simulink model "model"  (R2025b)
settings: Solver=ode1  StartTime=0.0  StopTime=Tstop  FixedStep=dt  RelTol=1e-3
undefined symbols (not defined in the file): d, N, opt_strategy, v0_vec, x0_vec
settings Model: Creator=Filippo  LastModifiedBy=dorec
settings DataIOCC: ReturnWorkspaceOutputs=off

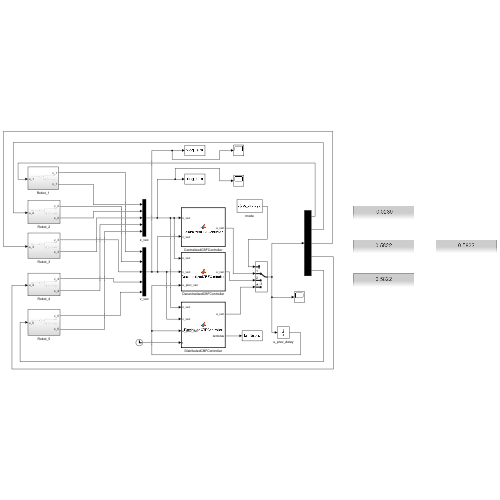
[thumbnail: Simulink's stored preview of the top-level diagram]
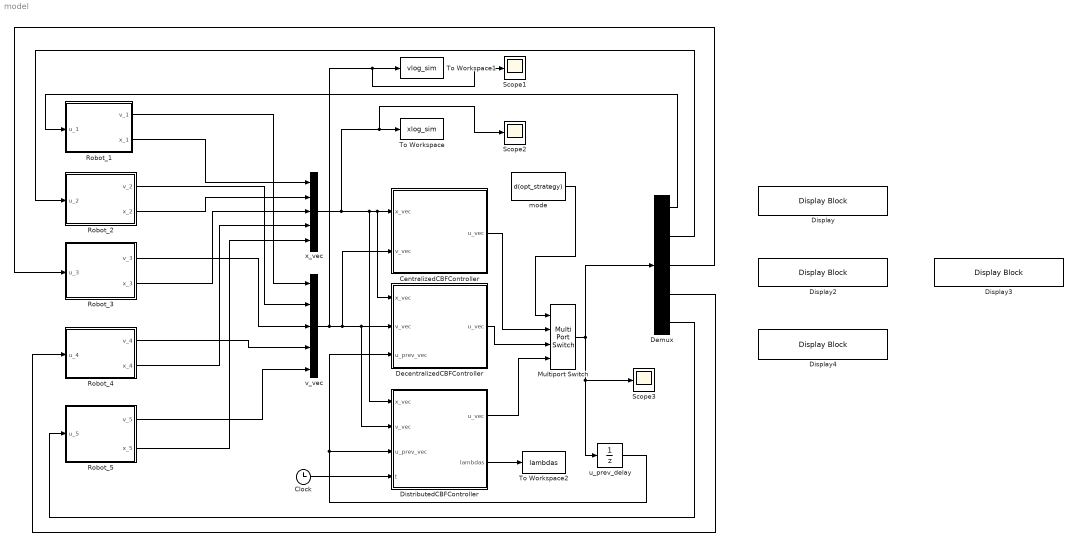
== system model ==
  CentralizedCBFController : MATLAB Function  TreatAsAtomicUnit=on
  Clock : Clock
  DecentralizedCBFController : MATLAB Function  TreatAsAtomicUnit=on
  Demux : Demux  Outputs=5
  Display{,2..4} (4 alike) : DisplayBlock  LabelPosition=Hide  Transparency=1  GridColor=[0.502, 0.502, 0.502]
  DistributedCBFController : MATLAB Function  TreatAsAtomicUnit=on
  Multiport Switch : MultiPortSwitch  SaturateOnIntegerOverflow=off  InputSameDT=off
  Robot_1 : Subsystem
  Robot_2 : Subsystem
  Robot_3 : Subsystem
  Robot_4 : Subsystem
  Robot_5 : Subsystem
  Scope1 : Scope
      settings: ActiveDisplayYMinimum=-1  ActiveDisplayYMaximum=1
  Scope2 : Scope
      settings: ActiveDisplayYMinimum=-11.952015322164979  ActiveDisplayYMaximum=12.436191131524438  DataLoggingVariableName=ScopeData2
  Scope3 : Scope
      settings: ActiveDisplayYMinimum=-11.952015322164979  ActiveDisplayYMaximum=12.436191131524438
  To Workspace : ToWorkspace  VariableName=xlog_sim  SampleTime=-1
  To Workspace1 : ToWorkspace  VariableName=vlog_sim  SampleTime=-1
  To Workspace2 : ToWorkspace  VariableName=lambdas  SampleTime=-1
  mode : Constant  Value=d(opt_strategy)
  u_prev_delay : UnitDelay  InitialCondition=zeros(2*N,1)  SampleTime=-1  HasFrameUpgradeWarning=on
  v_vec : Mux  Inputs=5
  x_vec : Mux  Inputs=5
  wires:
  CentralizedCBFController/1(u_vec) -> Multiport Switch/2
  u_prev_delay/1 -> DecentralizedCBFController/3(u_prev_vec), DistributedCBFController/3(u_prev_vec)
  mode/1 -> Multiport Switch/1
  Multiport Switch/1 -> Demux/1, Scope3/1, u_prev_delay/1
  DecentralizedCBFController/1(u_vec) -> Multiport Switch/3
  Robot_1/2(x_1) -> x_vec/1
  Robot_2/2(x_2) -> x_vec/2
  Robot_3/2(x_3) -> x_vec/3
  Robot_4/2(x_4) -> x_vec/4
  Robot_5/2(x_5) -> x_vec/5
  Robot_1/1(v_1) -> v_vec/1
  Robot_2/1(v_2) -> v_vec/2
  Robot_3/1(v_3) -> v_vec/3
  Robot_4/1(v_4) -> v_vec/4
  Robot_5/1(v_5) -> v_vec/5
  x_vec/1 -> Scope2/1, To Workspace/1, DistributedCBFController/1(x_vec), DecentralizedCBFController/1(x_vec), CentralizedCBFController/1(x_vec)
  v_vec/1 -> Scope1/1, To Workspace1/1, CentralizedCBFController/2(v_vec), DecentralizedCBFController/2(v_vec), DistributedCBFController/2(v_vec)
  Demux/5 -> Robot_5/1(u_5)
  Demux/1 -> Robot_1/1(u_1)
  Demux/4 -> Robot_4/1(u_4)
  Demux/3 -> Robot_3/1(u_3)
  Demux/2 -> Robot_2/1(u_2)
  Clock/1 -> DistributedCBFController/4(t)
  DistributedCBFController/1(u_vec) -> Multiport Switch/4
  DistributedCBFController/2(lambdas) -> To Workspace2/1

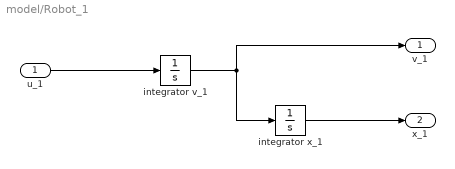
== system model/Robot_1 ==
  u_1 : Inport
  integrator v_1 : Integrator  InitialCondition=v0_vec(1:2)
  integrator x_1 : Integrator  InitialCondition=x0_vec(1:2)
  v_1 : Outport
  x_1 : Outport  Port=2
  wires:
  integrator v_1/1 -> v_1/1, integrator x_1/1
  u_1/1 -> integrator v_1/1
  integrator x_1/1 -> x_1/1

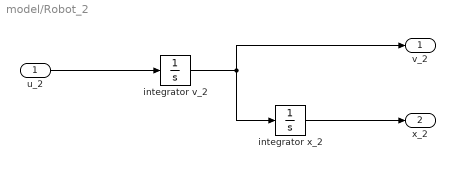
== system model/Robot_2 ==
  u_2 : Inport
  integrator v_2 : Integrator  InitialCondition=v0_vec(3:4)
  integrator x_2 : Integrator  InitialCondition=x0_vec(3:4)
  v_2 : Outport
  x_2 : Outport  Port=2
  wires:
  integrator v_2/1 -> v_2/1, integrator x_2/1
  u_2/1 -> integrator v_2/1
  integrator x_2/1 -> x_2/1

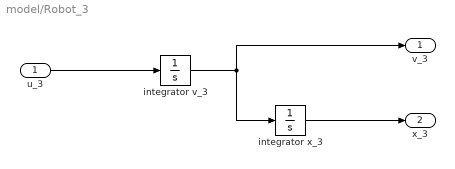
== system model/Robot_3 ==
  u_3 : Inport
  integrator v_3 : Integrator  InitialCondition=v0_vec(5:6)
  integrator x_3 : Integrator  InitialCondition=x0_vec(5:6)
  v_3 : Outport
  x_3 : Outport  Port=2
  wires:
  integrator v_3/1 -> v_3/1, integrator x_3/1
  u_3/1 -> integrator v_3/1
  integrator x_3/1 -> x_3/1

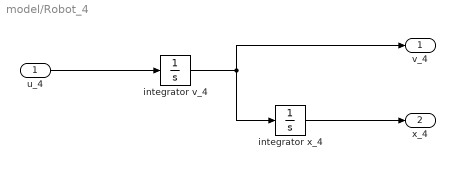
== system model/Robot_4 ==
  u_4 : Inport
  integrator v_4 : Integrator  InitialCondition=v0_vec(7:8)
  integrator x_4 : Integrator  InitialCondition=x0_vec(7:8)
  v_4 : Outport
  x_4 : Outport  Port=2
  wires:
  integrator v_4/1 -> v_4/1, integrator x_4/1
  u_4/1 -> integrator v_4/1
  integrator x_4/1 -> x_4/1

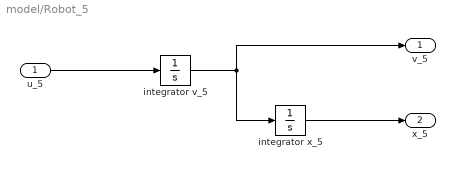
== system model/Robot_5 ==
  u_5 : Inport
  integrator v_5 : Integrator  InitialCondition=v0_vec(9:10)
  integrator x_5 : Integrator  InitialCondition=x0_vec(9:10)
  v_5 : Outport
  x_5 : Outport  Port=2
  wires:
  integrator v_5/1 -> v_5/1, integrator x_5/1
  u_5/1 -> integrator v_5/1
  integrator x_5/1 -> x_5/1

== matlab function model/DecentralizedCBFController ==
  data: x_vec input; u_vec output; v_vec input; u_prev_vec input
function u_vec = DecentralizedCBFController(x_vec, v_vec, u_prev_vec)
%#codegen
% Wrapper per chiamare decentralized_cbf_step da Simulink

coder.extrinsic('decentralized_cbf_step');

% Numero agenti (qui puoi fissare N=5 o leggere dal base workspace)
N = 5;                     % oppure usa evalin se vuoi:
% coder.extrinsic('evalin');
% N = evalin('base','N');

u_vec = zeros(2*N,1);      % per inferenza dimensioni

u_vec = decentralized_cbf_step(x_vec, v_vec, u_prev_vec);
end

== matlab function model/CentralizedCBFController ==
  data: x_vec input; u_vec output; v_vec input
function u_vec = CentralizedCBFController(x_vec, v_vec)
%#codegen
% Wrapper per chiamare la funzione esterna centralized_cbf_step
% dallo schema Simulink.

    coder.extrinsic('centralized_cbf_step');   % dico al coder che è una funzione MATLAB "normale"

    % Per permettere a Simulink di capire le dimensioni, prealloca u_vec
    % N = 5 --> 2N = 10. Se vuoi usare N dal workspace:
    %   coder.extrinsic('evalin');
    %   N = evalin('base','N');
    %   u_vec = zeros(2*N,1);
    N = 5;              % <-- se ora stai lavorando con 5 robot
    u_vec = zeros(2*N,1);

    % Chiamata vera e propria alla funzione di controllo
    u_vec = centralized_cbf_step(x_vec, v_vec);
end

== matlab function model/DistributedCBFController ==
  data: x_vec input; u_vec output; v_vec input; u_prev_vec input; t input; lambdas output
function [u_vec, lambdas] = DistributedCBFController(x_vec, v_vec, u_prev_vec, t)
%#codegen
% Wrapper per hybrid_cbf_step.m

coder.extrinsic('distributed_cbf_step');

% per inferenza dimensioni
N = 5;              % oppure leggi dal base workspace con evalin se vuoi
u_vec = zeros(2*N,1);
lambdas = zeros(4*N,1);
%vstdcon = zeros(2*N,1);

[u_vec, lambdas] = distributed_cbf_step(x_vec, v_vec, u_prev_vec, t);
end
